simulink model "joystick"  (R2023b)
settings: Solver=FixedStepAuto  StartTime=0.0  StopTime=inf  RelTol=1e-3  EnableMultiTasking=on
model workspace (MAT data in the model file):
  G = 2001
undefined symbols (not defined in the file): c_t, f_max, f_min, Kd, Kp, M, W
libraries: rpi_blkst x2
settings Model: ExtModeTrigDuration=2  Creator=yabde  LastModifiedBy=yabde
settings SolverCC: PositivePriorityOrder=on
settings OptimizationCC: EnhancedBackFolding=on  PassReuseOutputArgsAs=Individual arguments  ZeroExternalMemoryAtStartup=off  ZeroInternalMemoryAtStartup=off  MaxStackSize=64  OptimizeBlockOrder=speed  DifferentSizesBufferReuse=on  OptimizationCustomize=off  EfficientTunableParamExpr=on
settings DebuggingCC: ParameterTunabilityLossMsg=error
settings HardwareCC: ProdBitPerLong=64  ProdLargestAtomicInteger=LongLong  ProdLargestAtomicFloat=Double  ProdLongLongMode=on  ProdHWDeviceType=ARM Compatible->ARM 64-bit (LP64)
settings RTWCC: Description=Embedded Coder  SystemTargetFile=ert.tlc  HardwareBoard=Raspberry Pi (64bit)  TLCOptions="-aInlineSetEventsForThisBaseRateFcn=TLC_FALSE -aSuppressMultiTaskScheduler=TLC_FALSE  -aRateBasedStepFcn=0"  TemplateMakefile=ert_default_tmf  Toolchain=GNU GCC Embedded Linux  BuildConfiguration=Faster Runs
settings CodeAppCC: ForceParamTrailComments=on  IgnoreCustomStorageClasses=off  OperatorAnnotations=on  SimulinkDataObjDesc=on  SFDataObjDesc=on  InsertBlockDesc=on
settings ERTTargetCC: SupportVariableSizeSignals=on  ExtModeTransport=2  ExtModeStaticAlloc=on  ExtModeMexFile=ext_xcp  ExtModeIntrfLevel=Level2 - Open

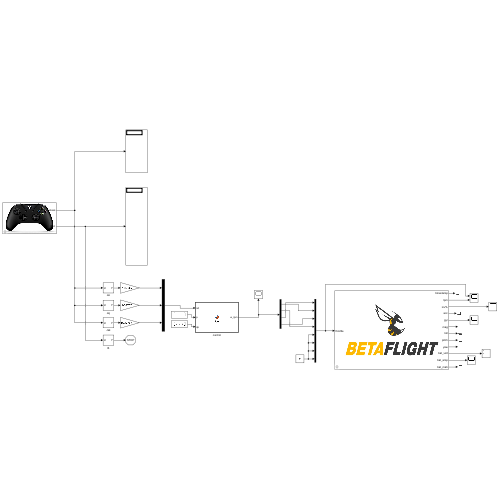
[thumbnail: Simulink's stored preview of the top-level diagram]
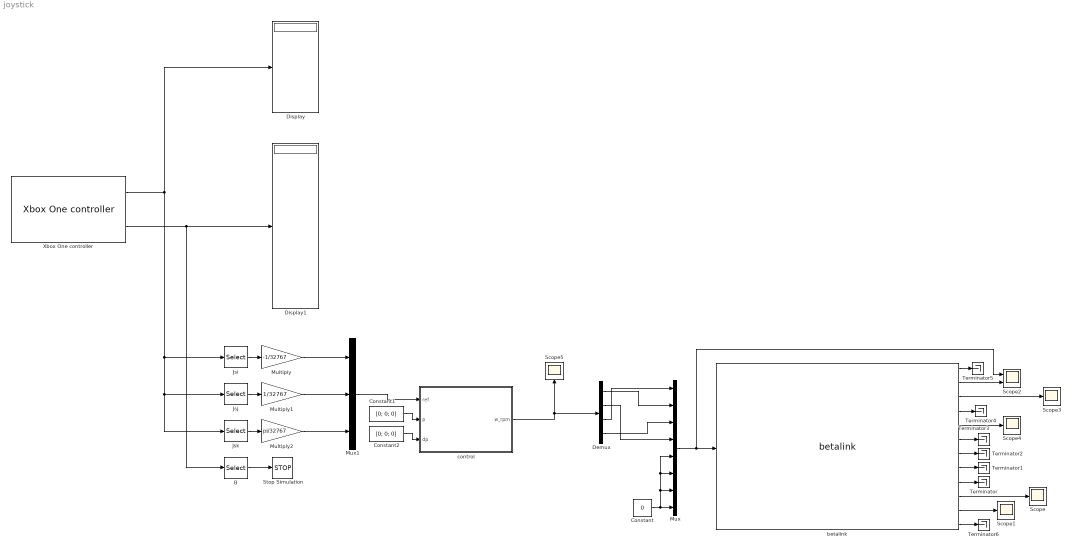
== system joystick ==
  B : Selector  IndexOptions=Index vector (dialog)  Indices=2  OutputSizes=1  RuntimeRangeChecks=on
  Constant : Constant  Value=0
  Constant1 : Constant  Value=[0; 0; 0]
  Constant2 : Constant  Value=[0; 0; 0]
  Demux : Demux
  Display : Display
  Display1 : Display
  Jsi : Selector  IndexOptions=Index vector (dialog)  Indices=2  OutputSizes=1  RuntimeRangeChecks=on
  Jsj : Selector  IndexOptions=Index vector (dialog)  Indices=1  OutputSizes=1  RuntimeRangeChecks=on
  Jsk : Selector  IndexOptions=Index vector (dialog)  Indices=4  OutputSizes=1  RuntimeRangeChecks=on
  Multiply : Gain  Gain=-1/32767
  Multiply1 : Gain  Gain=1/32767
  Multiply2 : Gain  Gain=pi/32767
  Mux : Mux  Inputs=8
  Mux1 : Mux  Inputs=3
  Scope{,1,3..5} (5 alike) : Scope
  Scope2 : Scope  NumInputPorts=2
  Stop Simulation : Stop
  Terminator{,1..6} (7 alike) : Terminator
  Xbox One controller : rpi_blkst/Xbox One controller  rpi_mask_ID=0  rpi_mask_Ts=0.01
      settings: SourceProductName=RPI Blockset
  betalink : rpi_blkst/betalink  rpi_mask_usb_serial_number=1042260556  rpi_mask_Ts=0.01
      settings: SourceProductName=RPI Blockset
  control : MATLAB Function  TreatAsAtomicUnit=on
  wires:
  Mux/1 -> betalink/1, Scope2/1
  Constant/1 -> Mux/5, Mux/6, Mux/7, Mux/8
  betalink/10 -> Scope/1
  betalink/11 -> Scope1/1
  betalink/2 -> Scope2/2
  betalink/3 -> Scope3/1
  betalink/5 -> Scope4/1
  betalink/9 -> Terminator/1
  betalink/8 -> Terminator1/1
  betalink/7 -> Terminator2/1
  betalink/6 -> Terminator3/1
  betalink/4 -> Terminator4/1
  betalink/12 -> Terminator6/1
  Xbox One controller/1 -> Jsk/1, Jsj/1, Jsi/1, Display/1
  betalink/1 -> Terminator5/1
  Jsj/1 -> Multiply1/1
  Jsk/1 -> Multiply2/1
  Constant1/1 -> control/2(p)
  Jsi/1 -> Multiply/1
  Multiply1/1 -> Mux1/2
  Multiply/1 -> Mux1/1
  Multiply2/1 -> Mux1/3
  Constant2/1 -> control/3(dp)
  control/1(w_rpm) -> Demux/1, Scope5/1
  Mux1/1 -> control/1(ref)
  Demux/1 -> Mux/2
  Demux/2 -> Mux/4
  Demux/3 -> Mux/1
  Demux/4 -> Mux/3
  B/1 -> Stop Simulation/1
  Xbox One controller/2 -> B/1, Display1/1

== matlab function joystick/control ==
  data: ref input; w_rpm output size=4; p input; dp input; Kp parameter; Kd parameter; M parameter; W parameter; c_t parameter; f_min parameter; f_max parameter
function w_rpm = fcn(ref,p,dp, Kp, Kd, M, W, c_t, f_min, f_max)

% Effort désiré
err = ref - p;
err(3) = wrapToPi(err(3));
tau = M * (Kp * err);
% tau = M * (-Kd * dp + Kp * err);

% --- QP formulation : min ||W_rot*f - tau||^2 + lambda||f||^2 ---
lambda = 1e-3;  % petit régularisateur
H = 2*(W'*W + lambda*eye(4));
f_qp = -2*W'*tau;
f0 = W \ tau;

% uniquement les bornes
options = optimoptions('quadprog','Display','off','Algorithm','active-set');
f = quadprog(H,f_qp,[],[],[],[],f_min,f_max,f0,options);

% Convertir en vitesses
w = sqrt(f ./ c_t);
w_rpm = w * 30/pi;

end
